simulink model "temp"  (R2015a)
settings: Solver=ode45  StartTime=0.0  StopTime=10.0  RelTol=1e-3
undefined symbols (not defined in the file): b_phi, b_x, Ke, Kt, l, La, m1, m2, Max_voltage, phi_0, r, Ra
settings Model: Creator=tvincent  LastModifiedBy=tvincent

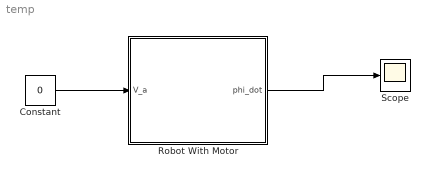
== system temp ==
  Constant : Constant  Value=0
  Robot With Motor : Subsystem
  Scope : Scope
  wires:
  Constant/1 -> Robot With Motor/1(V_a)
  Robot With Motor/1(phi_dot) -> Scope/1

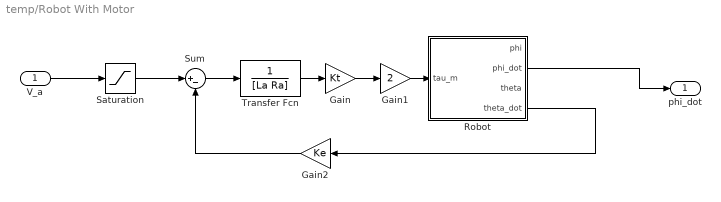
== system temp/Robot With Motor ==
  V_a : Inport
  Gain : Gain  Gain=Kt
  Gain1 : Gain  Gain=2
  Gain2 : Gain  Gain=Ke
  Robot : Subsystem
  Saturation : Saturate  UpperLimit=Max_voltage  LowerLimit=-Max_voltage
  Sum : Sum  Inputs=|+-
  Transfer Fcn : TransferFcn  Denominator=[La Ra]
  phi_dot : Outport
  wires:
  Robot/2(phi_dot) -> phi_dot/1
  Gain2/1 -> Sum/2
  Sum/1 -> Transfer Fcn/1
  Robot/4(theta_dot) -> Gain2/1
  Transfer Fcn/1 -> Gain/1
  Saturation/1 -> Sum/1
  V_a/1 -> Saturation/1
  Gain/1 -> Gain1/1
  Gain1/1 -> Robot/1(tau_m)

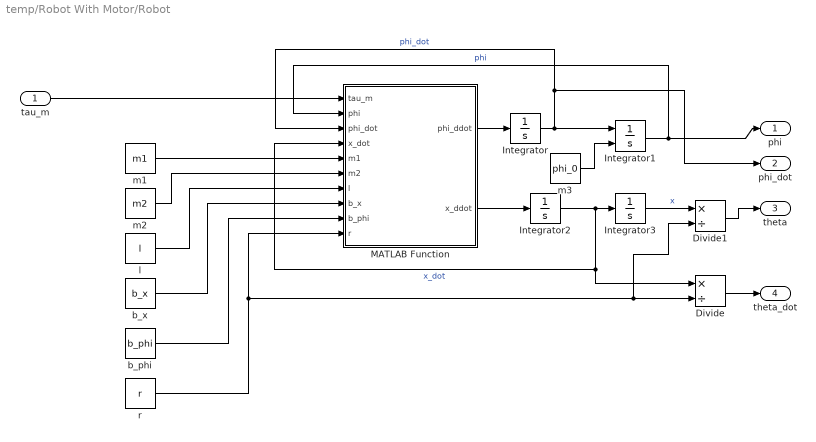
== system temp/Robot With Motor/Robot ==
  tau_m : Inport
  Divide : Product  Inputs=*/
  Divide1 : Product  Inputs=*/
  Integrator : Integrator
  Integrator1 : Integrator  InitialConditionSource=external  InitialCondition=pi
  Integrator2 : Integrator
  Integrator3 : Integrator
  MATLAB Function : MATLAB Function  TreatAsAtomicUnit=on
  b_phi : Constant  Value=b_phi
  b_x : Constant  Value=b_x
  l : Constant  Value=l
  m1 : Constant  Value=m1
  m2 : Constant  Value=m2
  m3 : Constant  Value=phi_0
  r : Constant  Value=r
  phi : Outport
  phi_dot : Outport  Port=2
  theta : Outport  Port=3
  theta_dot : Outport  Port=4
  wires:
  Integrator2/1 -> MATLAB Function/4(x_dot), Divide/1, Integrator3/1  "x_dot"
  m1/1 -> MATLAB Function/5(m1)
  Integrator1/1 -> phi/1, MATLAB Function/2(phi)  "phi"
  MATLAB Function/1(phi_ddot) -> Integrator/1
  MATLAB Function/2(x_ddot) -> Integrator2/1
  l/1 -> MATLAB Function/7(l)
  b_x/1 -> MATLAB Function/8(b_x)
  m2/1 -> MATLAB Function/6(m2)
  b_phi/1 -> MATLAB Function/9(b_phi)
  tau_m/1 -> MATLAB Function/1(tau_m)
  r/1 -> Divide1/2, Divide/2, MATLAB Function/10(r)
  Integrator/1 -> Integrator1/1, phi_dot/1, MATLAB Function/3(phi_dot)  "phi_dot"
  Divide/1 -> theta_dot/1
  Integrator3/1 -> Divide1/1  "x"
  Divide1/1 -> theta/1
  m3/1 -> Integrator1/2

== matlab function temp/Robot With Motor/Robot/MATLAB Function ==
  data: tau_m input; phi_ddot output; phi input; phi_dot input; x_dot input; m1 input; m2 input; l input; b_x input; b_phi input; r input; x_ddot output
function [phi_ddot,x_ddot] = phi_ddot(tau_m,phi,phi_dot,x_dot,m1,m2,l,b_x,b_phi,r)
%#codegen

g=9.81;

phi_ddot = ((g*(m1+m2) - m1*l*cos(phi)*(phi_dot)^2)*sin(phi) - cos(phi)*b_x*x_dot - ...
    ((m1+m2)/(m1*l))*b_phi*phi_dot + ((m1+m2)/(m1*l) + cos(phi)/r)*tau_m) / ...
    (l*(m2+m1*sin(phi)^2));

x_ddot = (g*m1*cos(phi)*sin(phi) - m1*l*sin(phi)*phi_dot^2 - b_x*x_dot - ...
    (cos(phi)/l)*b_phi*phi_dot + ((cos(phi)/l)+(1/r))*tau_m) / ...
    (m2+m1*sin(phi)^2);
